simulink model "sampleModel1712"  (R2023a)
settings: Solver=VariableStepAuto  StartTime=0.0  StopTime=10.0  RelTol=1e-3
libraries: hdlsllib x7, simulink x1
settings Model: Creator=user1  LastModifiedBy=user1

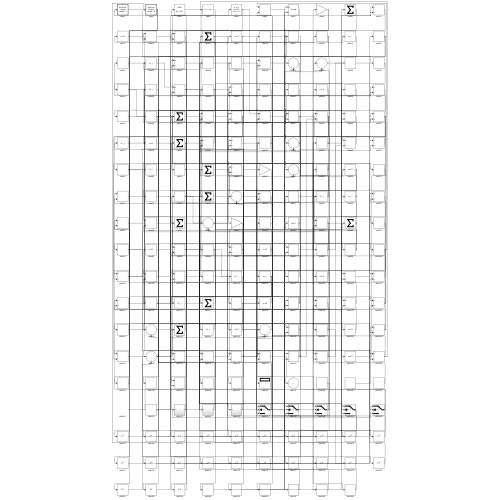
[thumbnail: Simulink's stored preview of the top-level diagram]
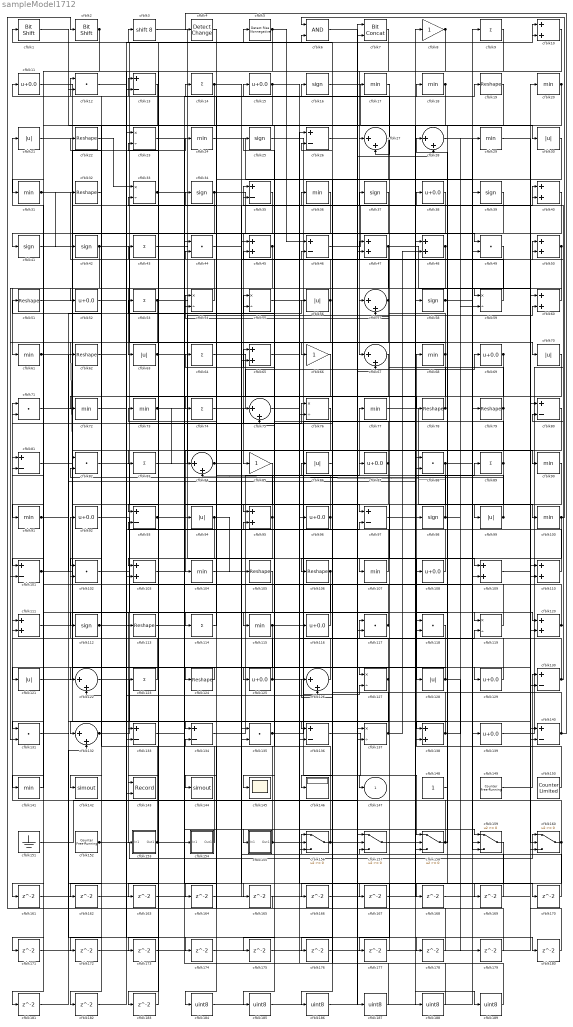
== system sampleModel1712 ==
  cfblk1 : hdlsllib/Logic and Bit Operations/Bit Shift  mode=Shift Left Logical  N=0
  cfblk{10,40,45,47..48,50,60,65,95,103,109..111,120,138} (15 alike) : Sum
  cfblk{17..18,20,24,29,31,36,61,68,72..73,77,90..91,100,104,107,115,141} (19 alike) : MinMax
  cfblk{13,26,35,46,80..81,93,97,101,130,133..134,136,140} (14 alike) : Sum  Inputs=+-
  cfblk{12,44,49,71,82,88,102,117..118,131,135} (11 alike) : DotProduct  OutDataTypeStr=Inherit: Inherit via internal rule
  cfblk{19,22,32,51,62,78..79,105..106,113,124} (11 alike) : Reshape
  cfblk{11,15,38,52,69,87,92,96,108,116,125,129,139} (13 alike) : Bias  Bias=0.0  SaturateOnIntegerOverflow=off
  cfblk{16,25,34,37,39,41..42,58,98,112} (10 alike) : Signum
  cfblk{9,14,43,53,64,74,83,89,114,123} (10 alike) : Sum  Inputs=+
  cfblk{23,33,54..55,59,76,119,127,137} (9 alike) : Product  Inputs=*/  RndMeth=Zero  SaturateOnIntegerOverflow=on
  cfblk{21,30,56,63,70,86,94,99,121,128} (10 alike) : Abs  SaturateOnIntegerOverflow=off
  cfblk{27..28,57,67,75,84,122,126,132} (9 alike) : Sum  Inputs=|++
  cfblk142 : ToWorkspace  VariableName=simout  SaveFormat=Timeseries  SampleTime=-1
  cfblk143 : Record  FileSettingsInternal="{\"entries\":[{\"content\":{\"excelSettings\":{\"content\":{},\"type\":\"Streamout.ExcelSettings\"}},\"type\":\"Streamout.FileSettingStorage\",\"uuid\":\"\"}],\"packageUris\":[\"http:\\/\\/schema.mathworks.com\\/mf0\\/streamout_blocks\\/R2020a\"],\"version\":\"1.0\"}"  Layout=[1 1]  SignalsInternal="{\"entries\":[{\"content\":{},\"type\":\"RecordBlkView.InputSignals\",\"uuid\":\"\"}],\"packageUris\":[\"http:\\/\\/schema.mathworks.com\\/mf0\\/streamout_blocks\\/R2020a\"],\"version\":\"1.0\"}"  VisualizationBindings="{\"xyplotplugin\":{\"info\":[{\"series\":[{\"bindingParametersList\":[{\"parameter\":\"X-Axis\",\"signalID\":3228,\"signalName\":\"cfblk8\"},{\"parameter\":\"Y-Axis\",\"signalID\":3232,\"signalName\":\"cfblk48\"}],\"seriesID\":35300}],\"subplotID\":1}]}}"  CompatibilityTag=XY  st=-1
  cfblk144 : ToWorkspace  VariableName=simout  SaveFormat=Timeseries  SampleTime=-1
  cfblk145 : Scope
  cfblk146 : Display
  cfblk148 : Constant  SampleTime=-1
  cfblk149 : hdlsllib/Sources/Counter Free-Running  NumBits=16  tsamp=-1
  cfblk150 : hdlsllib/Sources/Counter Limited  uplimit=7  tsamp=-1
  cfblk151 : Ground
  cfblk152 : hdlsllib/Sources/Counter Free-Running  NumBits=16  tsamp=-1
  cfblk153 : Subsystem
      settings: LibrarySourceBlock=|
      | hdlsllib/Ports &
      | Subsystems/Subsystem
  cfblk154 : Subsystem
      settings: LibrarySourceBlock=|
      | hdlsllib/Ports &
      | Subsystems/Subsystem
  cfblk155 : Subsystem
      settings: LibrarySourceBlock=|
      | hdlsllib/Ports &
      | Subsystems/Subsystem
  cfblk{156..160} (5 alike) : Switch  SaturateOnIntegerOverflow=off  InputSameDT=off
  cfblk{161..183} (23 alike) : Delay  SampleTime=1
  cfblk{184..189} (6 alike) : DataTypeConversion  OutDataTypeStr=uint8  SaturateOnIntegerOverflow=off  RndMeth=Floor
  cfblk2 : hdlsllib/Logic and Bit Operations/Bit Shift  mode=Shift Left Logical  N=0
  cfblk3 : ArithShift  BitShiftNumber=8
  cfblk4 : simulink/Logic and Bit Operations/Detect Change  vinit=0  OutDataTypeStr=boolean
      settings: LibrarySourceBlock=|
      | hdlsllib/Logic and Bit
      | Operations/Detect
      | Change
  cfblk5 : hdlsllib/Logic and Bit Operations/Detect Rise Nonnegative  vinit=0  OutDataTypeStr=boolean
  cfblk6 : Logic  AllPortsSameDT=off  OutDataTypeStr=boolean
  cfblk66 : Gain
  cfblk7 : hdlsllib/Logic and Bit Operations/Bit Concat  numInputs=2
  cfblk8 : Gain
  cfblk85 : Gain
  cfblk147 : Outport  VectorParamsAs1DForOutWhenUnconnected=off
  wires:
  cfblk158/1 -> cfblk71/1, cfblk28/1
  cfblk3/1 -> cfblk70/1
  cfblk16/1 -> cfblk30/1
  cfblk139/1 -> cfblk35/1
  cfblk31/1 -> cfblk49/1, cfblk42/1
  cfblk123/1 -> cfblk21/1
  cfblk150/1 -> cfblk68/1
  cfblk112/1 -> cfblk5/1, cfblk10/2
  cfblk60/1 -> cfblk59/1
  cfblk124/1 -> cfblk121/1
  cfblk55/1 -> cfblk147/1
  cfblk105/1 -> cfblk141/1
  cfblk109/1 -> cfblk20/1
  cfblk38/1 -> cfblk85/1
  cfblk24/1 -> cfblk139/1
  cfblk102/1 -> cfblk76/1
  cfblk22/1 -> cfblk33/1
  cfblk8/1 -> cfblk143/1, cfblk161/1
  cfblk121/1 -> cfblk24/1
  cfblk138/1 -> cfblk71/2, cfblk59/2
  cfblk76/1 -> cfblk145/1
  cfblk100/1 -> cfblk6/1, cfblk118/1, cfblk136/1
  cfblk77/1 -> cfblk99/1
  cfblk135/1 -> cfblk58/1, cfblk127/2
  cfblk44/1 -> cfblk40/1
  cfblk11/1 -> cfblk119/1
  cfblk107/1 -> cfblk13/1
  cfblk21/1 -> cfblk134/1
  cfblk81/1 -> cfblk97/1
  cfblk54/1 -> cfblk32/1
  cfblk134/1 -> cfblk77/1
  cfblk92/1 -> cfblk120/1
  cfblk80/1 -> cfblk104/1
  cfblk48/1 -> cfblk63/1, cfblk143/2, cfblk158/2
  cfblk98/1 -> cfblk73/1, cfblk84/2, cfblk29/1
  cfblk74/1 -> cfblk69/1
  cfblk70/1 -> cfblk106/1
  cfblk94/1 -> cfblk103/1, cfblk105/1
  cfblk23/1 -> cfblk155/1(In1)
  cfblk58/1 -> cfblk10/1, cfblk38/1
  cfblk127/1 -> cfblk46/2, cfblk182/1
  cfblk68/1 -> cfblk66/1, cfblk72/1, cfblk44/2
  cfblk25/1 -> cfblk98/1
  cfblk33/1 -> cfblk15/1, cfblk169/1, cfblk173/1
  cfblk111/1 -> cfblk34/1
  cfblk56/1 -> cfblk3/1, cfblk62/1
  cfblk154/1(Out1) -> cfblk111/1
  cfblk114/1 -> cfblk14/1
  cfblk49/1 -> cfblk78/1
  cfblk115/1 -> cfblk8/1, cfblk119/2, cfblk183/1
  cfblk46/1 -> cfblk40/2
  cfblk29/1 -> cfblk60/1
  cfblk83/1 -> cfblk60/2
  cfblk82/1 -> cfblk95/1
  cfblk5/1 -> cfblk13/2, cfblk46/1
  cfblk65/1 -> cfblk109/1
  cfblk148/1 -> cfblk156/1
  cfblk43/1 -> cfblk128/1
  cfblk9/1 -> cfblk67/1
  cfblk97/1 -> cfblk89/1
  cfblk116/1 -> cfblk75/1
  cfblk1/1 -> cfblk27/1
  cfblk17/1 -> cfblk27/2
  cfblk71/1 -> cfblk83/1
  cfblk62/1 -> cfblk76/2
  cfblk40/1 -> cfblk41/1
  cfblk88/1 -> cfblk100/1, cfblk107/1
  cfblk61/1 -> cfblk82/1, cfblk174/1
  cfblk152/1 -> cfblk160/1, cfblk97/2
  cfblk96/1 -> cfblk95/2, cfblk75/2
  cfblk132/1 -> cfblk39/1, cfblk126/2
  cfblk151/1 -> cfblk67/2
  cfblk110/1 -> cfblk25/1
  cfblk149/1 -> cfblk130/1
  cfblk66/1 -> cfblk156/2
  cfblk89/1 -> cfblk64/1, cfblk137/2
  cfblk119/1 -> cfblk37/1
  cfblk57/1 -> cfblk74/1, cfblk22/1
  cfblk129/1 -> cfblk81/1
  cfblk34/1 -> cfblk57/1, cfblk133/2
  cfblk18/1 -> cfblk115/1, cfblk138/2
  cfblk27/1 -> cfblk146/1
  cfblk53/1 -> cfblk140/1, cfblk131/2
  cfblk30/1 -> cfblk94/1
  cfblk126/1 -> cfblk92/1
  cfblk106/1 -> cfblk153/1(In1), cfblk156/3
  cfblk69/1 -> cfblk138/1, cfblk125/1
  cfblk59/1 -> cfblk35/2
  cfblk95/1 -> cfblk113/1, cfblk33/2
  cfblk125/1 -> cfblk129/1, cfblk43/1, cfblk140/2
  cfblk160/1 -> cfblk47/1, cfblk118/2, cfblk177/1
  cfblk51/1 -> cfblk17/1
  cfblk140/1 -> cfblk4/1, cfblk102/2
  cfblk133/1 -> cfblk56/1
  cfblk73/1 -> cfblk159/1, cfblk84/1, cfblk159/3
  cfblk118/1 -> cfblk131/1
  cfblk99/1 -> cfblk86/1, cfblk82/2
  cfblk15/1 -> cfblk116/1, cfblk65/2
  cfblk64/1 -> cfblk108/1
  cfblk37/1 -> cfblk132/1
  cfblk87/1 -> cfblk144/1, cfblk53/1
  cfblk2/1 -> cfblk31/1, cfblk12/2
  cfblk130/1 -> cfblk23/2, cfblk50/1
  cfblk120/1 -> cfblk80/2, cfblk81/2
  cfblk85/1 -> cfblk114/1
  cfblk63/1 -> cfblk133/1, cfblk90/1
  cfblk103/1 -> cfblk18/1
  cfblk91/1 -> cfblk54/1, cfblk136/2
  cfblk36/1 -> cfblk102/1
  cfblk113/1 -> cfblk19/1
  cfblk155/1(Out1) -> cfblk12/1, cfblk117/1
  cfblk6/1 -> cfblk157/1
  cfblk101/1 -> cfblk124/1, cfblk88/2
  cfblk10/1 -> cfblk101/1
  cfblk50/1 -> cfblk61/1, cfblk186/1
  cfblk14/1 -> cfblk117/2, cfblk181/1
  cfblk86/1 -> cfblk16/1
  cfblk84/1 -> cfblk50/2, cfblk167/1
  cfblk45/1 -> cfblk93/1, cfblk91/1
  cfblk156/1 -> cfblk55/2, cfblk51/1, cfblk28/2, cfblk178/1
  cfblk104/1 -> cfblk135/2
  cfblk42/1 -> cfblk88/1, cfblk96/1, cfblk101/2
  cfblk108/1 -> cfblk55/1
  cfblk72/1 -> cfblk127/1
  cfblk41/1 -> cfblk154/1(In1)
  cfblk79/1 -> cfblk159/2, cfblk54/2
  cfblk122/1 -> cfblk160/2
  cfblk128/1 -> cfblk122/1, cfblk179/1
  cfblk47/1 -> cfblk110/1, cfblk176/1
  cfblk136/1 -> cfblk158/1
  cfblk13/1 -> cfblk52/1
  cfblk12/1 -> cfblk123/1
  cfblk32/1 -> cfblk142/1
  cfblk20/1 -> cfblk171/1, cfblk172/1
  cfblk141/1 -> cfblk111/2
  cfblk28/1 -> cfblk79/1
  cfblk117/1 -> cfblk65/1, cfblk112/1
  cfblk137/1 -> cfblk87/1, cfblk48/2, cfblk1/1
  cfblk93/1 -> cfblk130/2, cfblk158/3
  cfblk153/1(Out1) -> cfblk36/1, cfblk122/2
  cfblk78/1 -> cfblk45/2, cfblk11/1
  cfblk161/1 -> cfblk45/1
  cfblk39/1 -> cfblk162/1
  cfblk162/1 -> cfblk103/2
  cfblk35/1 -> cfblk163/1
  cfblk163/1 -> cfblk49/2
  cfblk4/1 -> cfblk164/1
  cfblk164/1 -> cfblk137/1
  cfblk131/1 -> cfblk165/1
  cfblk165/1 -> cfblk2/1
  cfblk159/1 -> cfblk166/1
  cfblk166/1 -> cfblk48/1
  cfblk19/1 -> cfblk168/1
  cfblk168/1 -> cfblk120/2
  cfblk169/1 -> cfblk6/2
  cfblk75/1 -> cfblk170/1
  cfblk170/1 -> cfblk135/1
  cfblk171/1 -> cfblk109/2
  cfblk172/1 -> cfblk47/2
  cfblk173/1 -> cfblk160/3
  cfblk174/1 -> cfblk110/2
  cfblk67/1 -> cfblk175/1
  cfblk175/1 -> cfblk157/2
  cfblk176/1 -> cfblk126/1
  cfblk177/1 -> cfblk157/3
  cfblk178/1 -> cfblk57/2
  cfblk179/1 -> cfblk134/2
  cfblk52/1 -> cfblk180/1
  cfblk180/1 -> cfblk80/1
  cfblk181/1 -> cfblk132/2
  cfblk182/1 -> cfblk23/1
  cfblk183/1 -> cfblk93/2
  cfblk7/1 -> cfblk184/1
  cfblk184/1 -> cfblk9/1
  cfblk90/1 -> cfblk185/1
  cfblk185/1 -> cfblk7/1
  cfblk186/1 -> cfblk7/2
  cfblk26/1 -> cfblk187/1
  cfblk187/1 -> cfblk44/1
  cfblk167/1 -> cfblk188/1
  cfblk188/1 -> cfblk26/1
  cfblk157/1 -> cfblk189/1
  cfblk189/1 -> cfblk26/2

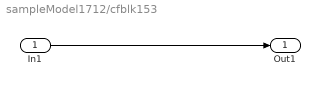
== system sampleModel1712/cfblk153 ==
  In1 : Inport
  Out1 : Outport
  wires:
  In1/1 -> Out1/1

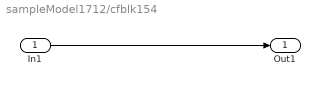
== system sampleModel1712/cfblk154 ==
  In1 : Inport
  Out1 : Outport
  wires:
  In1/1 -> Out1/1

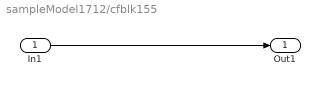
== system sampleModel1712/cfblk155 ==
  In1 : Inport
  Out1 : Outport
  wires:
  In1/1 -> Out1/1
